simulink model "example_trajectory"  (R2016a)
settings: Solver=VariableStepAuto  StartTime=0.0  StopTime=30.0  RelTol=1e-3
settings Model: Creator=mgreiff  LastModifiedBy=mgreiff

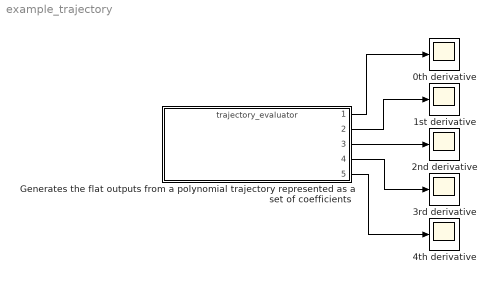
== system example_trajectory ==
  0th derivative : Scope
  1st derivative : Scope
  2nd derivative : Scope
  3rd derivative : Scope
  4th derivative : Scope
  Generates the flat outputs from a polynomial trajectory represented as a set of coefficients : ModelReference  ModelNameDialog=trajectory_evaluator.slx  SimulationMode=Normal  ModelReferenceVersion=1.106
  wires:
  Generates the flat outputs from a polynomial trajectory represented as a set of coefficients/3 -> 2nd derivative/1
  Generates the flat outputs from a polynomial trajectory represented as a set of coefficients/4 -> 3rd derivative/1
  Generates the flat outputs from a polynomial trajectory represented as a set of coefficients/5 -> 4th derivative/1
  Generates the flat outputs from a polynomial trajectory represented as a set of coefficients/2 -> 1st derivative/1
  Generates the flat outputs from a polynomial trajectory represented as a set of coefficients/1 -> 0th derivative/1
